simulink model "vibration_fault_model"  (R2026a)
settings: Solver=VariableStepAuto  StopTime=300
undefined symbols (not defined in the file): engine
settings Model: LastModifiedBy=GOD

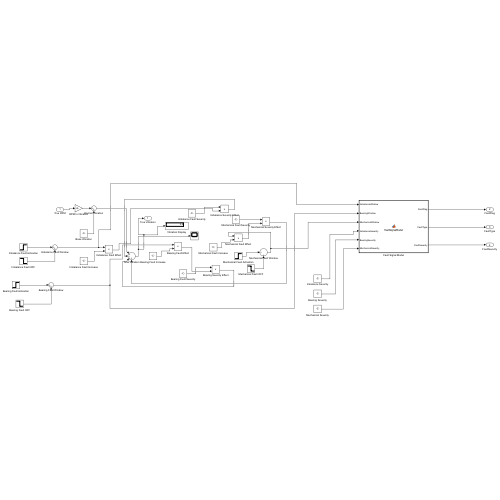
[thumbnail: Simulink's stored preview of the top-level diagram]
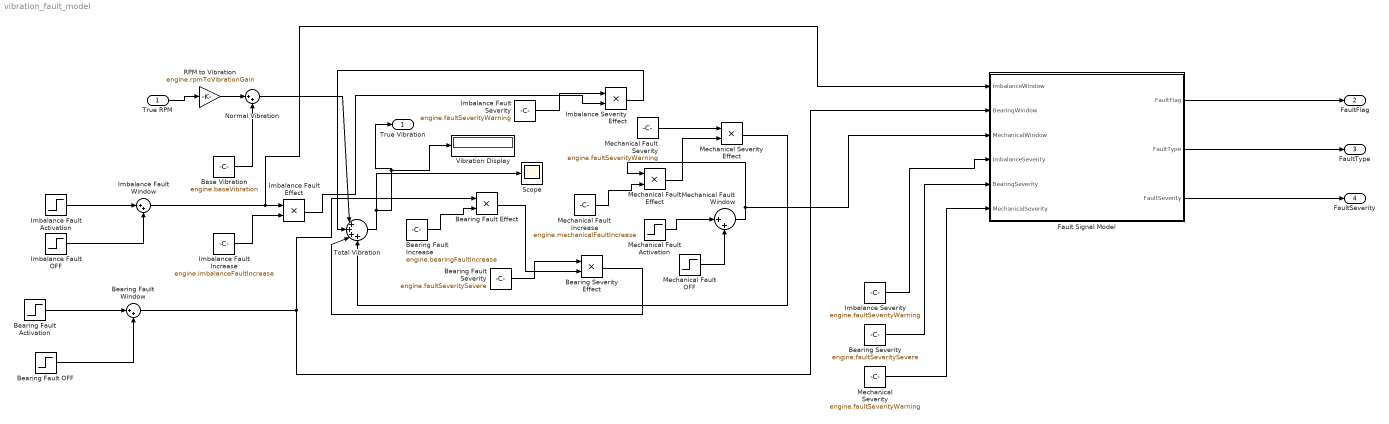
== system vibration_fault_model ==
  True RPM : Inport
  Base Vibration : Constant  Value=engine.baseVibration
  Bearing Fault Activation : Step  Time=180  SampleTime=0
  Bearing Fault Effect : Product
  Bearing Fault Increase : Constant  Value=engine.bearingFaultIncrease
  Bearing Fault OFF : Step  Time=240  FinalValue=-1  SampleTime=0
  Bearing Fault Severity : Constant  Value=engine.faultSeveritySevere
  Bearing Fault Window : Sum  Inputs=|++
  Bearing Severity : Constant  Value=engine.faultSeveritySevere
  Bearing Severity Effect : Product
  Fault Signal Model : MATLAB Function  TreatAsAtomicUnit=on
  Imbalance Fault Activation : Step  Time=100  SampleTime=0
  Imbalance Fault Effect : Product
  Imbalance Fault Increase : Constant  Value=engine.imbalanceFaultIncrease
  Imbalance Fault OFF : Step  Time=180  FinalValue=-1  SampleTime=0
  Imbalance Fault Severity : Constant  Value=engine.faultSeverityWarning
  Imbalance Fault Window : Sum  Inputs=|++
  Imbalance Severity : Constant  Value=engine.faultSeverityWarning
  Imbalance Severity Effect : Product
  Mechanical Fault Activation : Step  Time=240  SampleTime=0
  Mechanical Fault Effect : Product
  Mechanical Fault Increase : Constant  Value=engine.mechanicalFaultIncrease
  Mechanical Fault OFF : Step  Time=300  FinalValue=-1  SampleTime=0
  Mechanical Fault Severity : Constant  Value=engine.faultSeverityWarning
  Mechanical Fault Window : Sum  Inputs=|++
  Mechanical Severity : Constant  Value=engine.faultSeverityWarning
  Mechanical Severity Effect : Product
  Normal Vibration : Sum  Inputs=|++
  RPM to Vibration : Gain  Gain=engine.rpmToVibrationGain
  Scope : Scope
      settings: ActiveDisplayYMinimum=1.5125  ActiveDisplayYMaximum=3.3875
  Total Vibration : Sum  Inputs=|++++
  Vibration Display : Display
  True Vibration : Outport
  FaultFlag : Outport  Port=2
  FaultType : Outport  Port=3
  FaultSeverity : Outport  Port=4
  wires:
  RPM to Vibration/1 -> Normal Vibration/1
  Base Vibration/1 -> Normal Vibration/2
  Imbalance Fault Increase/1 -> Imbalance Fault Effect/2
  Normal Vibration/1 -> Total Vibration/1
  Total Vibration/1 -> True Vibration/1, Vibration Display/1, Scope/1
  Bearing Fault Increase/1 -> Bearing Fault Effect/2
  Mechanical Fault Increase/1 -> Mechanical Fault Effect/2
  Imbalance Fault Effect/1 -> Imbalance Severity Effect/2
  Imbalance Fault Severity/1 -> Imbalance Severity Effect/1
  Imbalance Severity Effect/1 -> Total Vibration/2
  Bearing Fault Severity/1 -> Bearing Severity Effect/1
  Bearing Fault Effect/1 -> Bearing Severity Effect/2
  Bearing Severity Effect/1 -> Total Vibration/3
  Mechanical Fault Severity/1 -> Mechanical Severity Effect/1
  Mechanical Fault Effect/1 -> Mechanical Severity Effect/2
  Mechanical Severity Effect/1 -> Total Vibration/4
  Imbalance Fault Activation/1 -> Imbalance Fault Window/1
  Imbalance Fault OFF/1 -> Imbalance Fault Window/2
  Imbalance Fault Window/1 -> Fault Signal Model/1(ImbalanceWindow), Imbalance Fault Effect/1
  Bearing Fault Activation/1 -> Bearing Fault Window/1
  Bearing Fault OFF/1 -> Bearing Fault Window/2
  Mechanical Fault Activation/1 -> Mechanical Fault Window/1
  Mechanical Fault OFF/1 -> Mechanical Fault Window/2
  Mechanical Fault Window/1 -> Fault Signal Model/3(MechanicalWindow), Mechanical Fault Effect/1
  True RPM/1 -> RPM to Vibration/1
  Imbalance Severity/1 -> Fault Signal Model/4(ImbalanceSeverity)
  Bearing Severity/1 -> Fault Signal Model/5(BearingSeverity)
  Mechanical Severity/1 -> Fault Signal Model/6(MechanicalSeverity)
  Bearing Fault Window/1 -> Fault Signal Model/2(BearingWindow), Bearing Fault Effect/1
  Fault Signal Model/3(FaultSeverity) -> FaultSeverity/1
  Fault Signal Model/2(FaultType) -> FaultType/1
  Fault Signal Model/1(FaultFlag) -> FaultFlag/1

== matlab function vibration_fault_model/Fault Signal Model ==
  data: ImbalanceWindow input; FaultFlag output; BearingWindow input; MechanicalWindow input; ImbalanceSeverity input; BearingSeverity input; MechanicalSeverity input; FaultType output; FaultSeverity output
function [FaultFlag, FaultType, FaultSeverity] = FaultSignalModel(...
    ImbalanceWindow, BearingWindow, MechanicalWindow, ...
    ImbalanceSeverity, BearingSeverity, MechanicalSeverity)
% Converts the three existing fault-activation windows (0/1 signals,
% already built inside vibration_fault_model.slx) into the project's
% standard FaultFlag/FaultType/FaultSeverity signals.
% FaultType encoding: 0 = none, 1 = Imbalance, 2 = Bearing, 3 = Mechanical.
% If windows overlap, priority order is Mechanical > Bearing > Imbalance.
if MechanicalWindow >= 0.5
    FaultFlag = 1; FaultType = 3; FaultSeverity = MechanicalSeverity;
elseif BearingWindow >= 0.5
    FaultFlag = 1; FaultType = 2; FaultSeverity = BearingSeverity;
elseif ImbalanceWindow >= 0.5
    FaultFlag = 1; FaultType = 1; FaultSeverity = ImbalanceSeverity;
else
    FaultFlag = 0; FaultType = 0; FaultSeverity = 0;
end
end
